simulink model "system_blocks_lqr_servo"  (R2019b)
settings: Solver=ode4  StartTime=t_start  StopTime=t_stop  FixedStep=t_step  RelTol=1e-3
undefined symbols (not defined in the file or in its folder): Ap, Bp, Cp, Dp, Gr, Gy, Gz
settings Model: Creator=Vish  LastModifiedBy=Vish

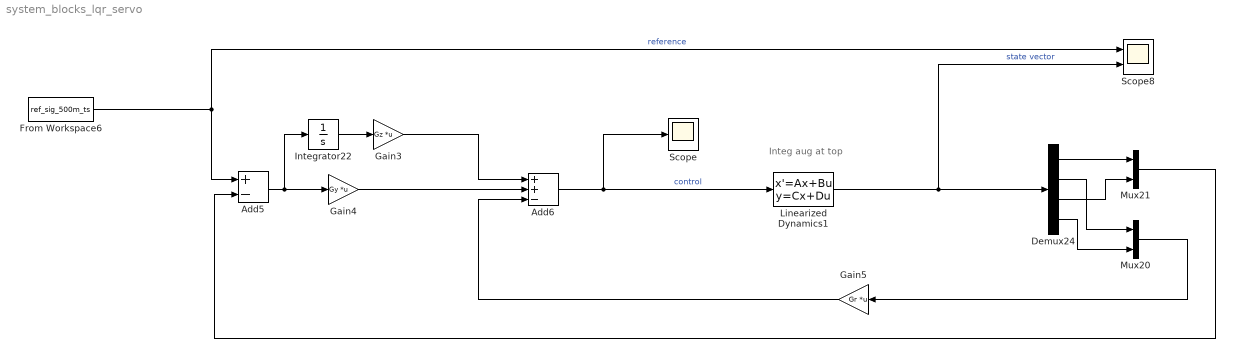
== system system_blocks_lqr_servo ==
  note: Integ aug at top
  Add5 : Sum  Inputs=+-
  Add6 : Sum  Inputs=++-
  Demux24 : Demux
  From Workspace6 : FromWorkspace  VariableName=ref_sig_500m_ts  SampleTime=0
  Gain3 : Gain  Gain=Gz  Multiplication=Matrix(K*u)
  Gain4 : Gain  Gain=Gy  Multiplication=Matrix(K*u)
  Gain5 : Gain  Gain=Gr  Multiplication=Matrix(K*u)
  Integrator22 : Integrator
  Linearized Dynamics1 : StateSpace  A=Ap  B=Bp  C=Cp  D=Dp  InitialCondition=[-3,0,0,0]
  Mux20 : Mux  Inputs=2
  Mux21 : Mux  Inputs=2
  Scope : Scope
  Scope8 : Scope  NumInputPorts=2
  wires:
  Demux24/3 -> Mux21/2
  Mux21/1 -> Add5/2
  Add5/1 -> Gain4/1, Integrator22/1
  Demux24/1 -> Mux21/1
  Demux24/4 -> Mux20/2
  Add6/1 -> Scope/1, Linearized Dynamics1/1  "control"
  Linearized Dynamics1/1 -> Scope8/2, Demux24/1  "state vector"
  From Workspace6/1 -> Scope8/1, Add5/1  "reference"
  Integrator22/1 -> Gain3/1
  Gain3/1 -> Add6/1
  Gain4/1 -> Add6/2
  Demux24/2 -> Mux20/1
  Mux20/1 -> Gain5/1
  Gain5/1 -> Add6/3
